simulink library "simviewers"  (Simulink 6.0)
settings: Solver=ode45  SolverMode=SingleTasking  StartTime=0.0  StopTime=10.0  RelTol=1e-3
model workspace (MAT data in the model file):
  libCache.blocksTree = {{'simviewers', {'Floating Scope'; 'Scope'; 'XY Graph'}}}
  libCache.blockNames{1} = 'simviewers'
  libCache.blockNames{2} = 'simviewers/Floating
    | Scope'
  libCache.blockNames{3} = 'simviewers/Scope'
  libCache.blockNames{4} = 'simviewers/XY Graph'
undefined symbols (not defined in the file or in its folder): sfunxy
PreSaveFcn:
  | iomanager('UpdateCache',bdroot(gcs))
settings Model: LibraryType=IOLibrary  Creator=howie  LastModifiedBy=howie  ExtModeAutoUpdateStatusClock=off  ProdHWDeviceType=Specified
settings OptimizationCC: BooleanDataType=off
settings DebuggingCC: CheckExecutionContextPreStartOutputMsg=on  CheckExecutionContextRuntimeOutputMsg=on  SolverPrmCheckMsg=none
settings HardwareCC: ProdHWDeviceType=Specified  TargetUnknown=on
settings SFSimCC: SFSimApplyToAllLibs=on  SFSimBuildMode=Incremental

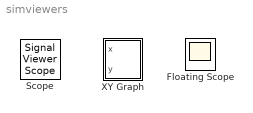
== system simviewers ==
  Floating Scope : Scope
      settings: Floating=on
  Scope : SignalViewerScope  IOType=viewer  RefreshTime=0.035000
  XY Graph : Subsystem  IOType=viewer  LoadFcn=sfunxy([],[],[],'LoadBlock')  StartFcn=sfunxy([],[],[],'Start')  StopFcn=sfunxy([],[],[],'Stop')  TreatAsAtomicUnit=on  PropExecContextAcrossSSBoundary=on  SimViewingDevice=on  mask(XY scope.){xmin=-1, xmax=1, ymin=-1, ymax=1, st=-1}
      mask prompts: xmin "x-min:"; xmax "x-max:"; ymin "y-min:"; ymax "y-max:"; st "Sample time:"
      mask help: XY scope using MATLAB graph window. First input is used as time base. Enter plotting ranges.
      settings: CopyFcn=sfunxy([],[],[],'CopyBlock')  DeleteFcn=sfunxy([],[],[],'DeleteBlock')  NameChangeFcn=sfunxy([],[],[],'NameChange')
      mask Help: This block can be used to explore limit cycles. Look at the m-file sfunxy.m to see how it works.
      mask Display: plot([.05 .95 .95 .05 .05],[.45 .45 .95 .95 .45], 0.5+cos(0:0.1:2*pi)*0.3,0.7+sin(0:0.1:2*pi)*0.2)

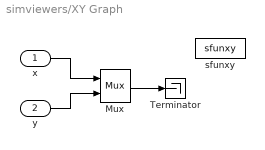
== system simviewers/XY Graph ==
  x : Inport  LatchInput=off
  y : Inport  Port=2  LatchInput=off
  Mux : Mux  Inputs=2
  Terminator : Terminator
  sfunxy : S-Function  IOType=viewer  FunctionName=sfunxy  Parameters=[xmin xmax ymin ymax], st
  wires:
  y/1 -> Mux/2
  x/1 -> Mux/1
  Mux/1 -> Terminator/1
